simulink model "Lab3_Bai3"  (R2019a)
settings: Solver=VariableStepAuto  StartTime=0.0  StopTime=10.0  RelTol=1e-3
settings Model: Creator=ASUS  LastModifiedBy=ASUS

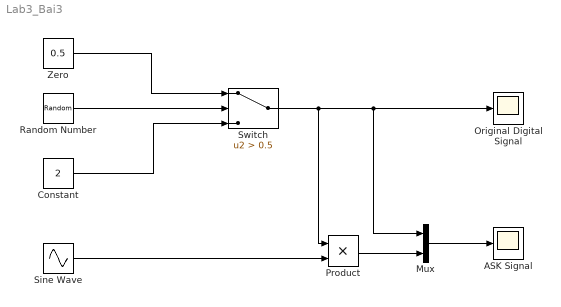
== system Lab3_Bai3 ==
  ASK Signal : Scope
  Constant : Constant  Value=2
  Mux : Mux  Inputs=2
  Original Digital Signal : Scope
  "Product " : Product
  "Random Number " : RandomNumber  SampleTime=0.1
  Sine Wave : Sin  Frequency=100  SampleTime=0.001
  "Switch " : Switch  Criteria=u2 > Threshold  Threshold=0.5
  Zero : Constant  Value=0.5  OutDataTypeStr=Inherit: Inherit via back propagation
  wires:
  Constant/1 -> "Switch "/3
  "Random Number "/1 -> "Switch "/2
  Zero/1 -> "Switch "/1
  "Switch "/1 -> "Product "/1, Mux/1, Original Digital Signal/1
  "Product "/1 -> Mux/2
  Mux/1 -> ASK Signal/1
  Sine Wave/1 -> "Product "/2
